simulink model "ridmasimulink"  (R2019b)
settings: Solver=VariableStepAuto  StartTime=0.0  StopTime=10.0  RelTol=1e-3
values from neighbouring files (symbols this model uses):
  A = [0 0 1 0 ... (first row only)    [RIP_ABCD_SS.m]    (also in RIP_ABCD_SS_1.m; RIP_ABCD_SS_2.m = [0   0    1   0; RIP_ABCD_SS_3.m; RIP_ABCD_SS_POLE_PLACE.m)
  B = Kg * kt * B / Rm    [RIP_ABCD_SS.m]    (also in RIP_ABCD_SS_1.m; RIP_ABCD_SS_2.m; RIP_ABCD_SS_3.m; RIP_ABCD_SS_POLE_PLACE.m)
  C = eye(2,4)    [RIP_ABCD_SS.m]    (also in RIP_ABCD_SS_1.m; RIP_ABCD_SS_2.m = [1 0 0 0; RIP_ABCD_SS_3.m; RIP_ABCD_SS_POLE_PLACE.m)
  D = zeros(2,1)    [RIP_ABCD_SS.m]    (also in RIP_ABCD_SS_1.m; RIP_ABCD_SS_2.m = [0; RIP_ABCD_SS_3.m; RIP_ABCD_SS_POLE_PLACE.m)
  K = [0 0 0 0]    [Pole_placement.m]    (also in RIP_ABCD_SS.m = lqr(A,B,Q,R); RIP_ABCD_SS_POLE_PLACE.m = lqr(A,B,Q,R); ripbalanced.m = acker(A,B,DP); setup_rotpen.m = d_balance(A, B, zeta, wn, p3, p4))
libraries: simulink_extras x3
settings Model: Creator=Ridma  LastModifiedBy=Ridma

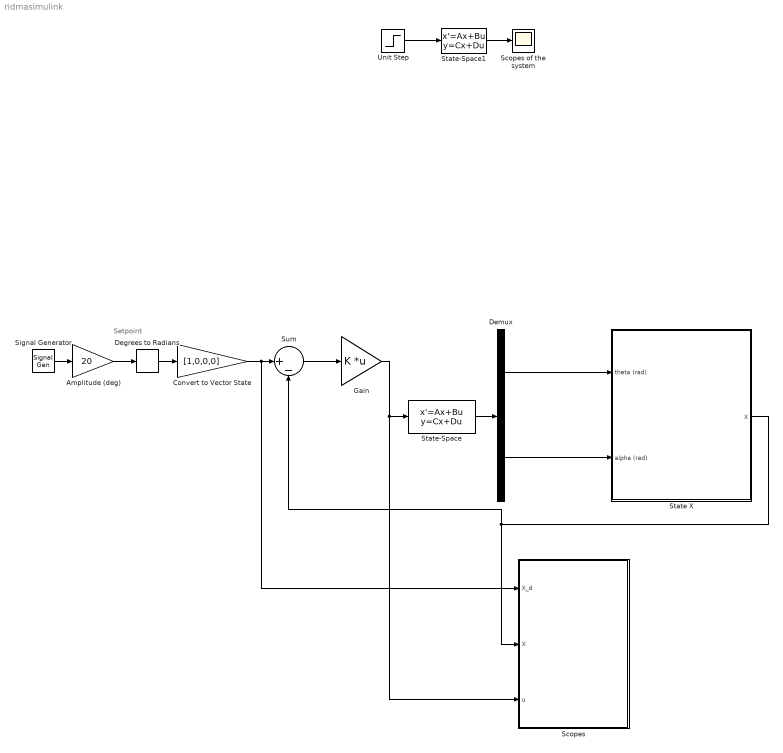
== system ridmasimulink ==
  note: Setpoint
  " State X " : Subsystem
      mask Display: image('$imagefile'); % Use "Edit Image" on toolstrip to change.
  Amplitude (deg) : Gain  Gain=20  SaturateOnIntegerOverflow=on  OutDataTypeStr=Inherit: Same as input  ParamDataTypeStr=Inherit: Same as input
  Convert to Vector State : Gain  Gain=[1,0,0,0]
  Degrees to Radians : simulink_extras/Transformations/Degrees to Radians
  Demux : Demux  Outputs=2
  Gain : Gain  Gain=K  Multiplication=Matrix(K*u)
  Scopes : Subsystem
  Scopes of the system : Scope
  Signal Generator : SignalGenerator  WaveForm=square  Frequency=0.1
  State-Space : StateSpace  A=A  B=B  C=C  D=D  InitialCondition=0
  State-Space1 : StateSpace  A=A  B=B  C=C  D=D  InitialCondition=0
  Sum : Sum  Inputs=|+-
  Unit Step : Step  SampleTime=0
  wires:
  Demux/2 -> " State X "/2(alpha (rad))
  Demux/1 -> " State X "/1(theta (rad))
  State-Space/1 -> Demux/1
  Amplitude (deg)/1 -> Degrees to Radians/1
  Degrees to Radians/1 -> Convert to Vector State/1
  Signal Generator/1 -> Amplitude (deg)/1
  Convert to Vector State/1 -> Scopes/1(X_d), Sum/1
  Sum/1 -> Gain/1
  Gain/1 -> Scopes/3(u), State-Space/1
  " State X "/1(X) -> Sum/2, Scopes/2(X)
  Unit Step/1 -> State-Space1/1
  State-Space1/1 -> Scopes of the system/1

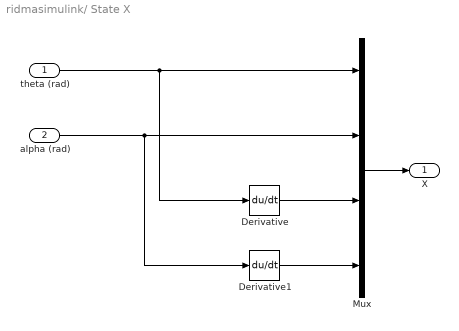
== system ridmasimulink/ State X  ==
  theta (rad) : Inport
  alpha (rad) : Inport  Port=2
  Derivative : Derivative
  Derivative1 : Derivative
  Mux : Mux
  X : Outport  VectorParamsAs1DForOutWhenUnconnected=off
  wires:
  alpha (rad)/1 -> Derivative1/1, Mux/2
  Mux/1 -> X/1
  theta (rad)/1 -> Derivative/1, Mux/1
  Derivative/1 -> Mux/3
  Derivative1/1 -> Mux/4

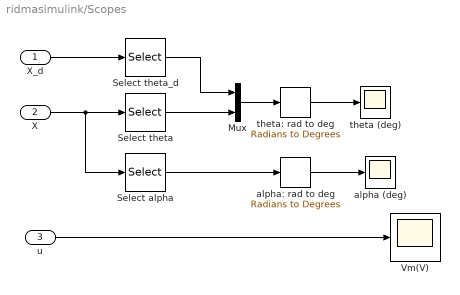
== system ridmasimulink/Scopes ==
  X_d : Inport
  X : Inport  Port=2
  u : Inport  Port=3
  Mux : Mux  Inputs=2
  Select alpha : Selector  InputPortWidth=4  IndexOptions=Index vector (dialog)  Indices=2  OutputSizes=[(-2)]
  Select theta : Selector  InputPortWidth=4  IndexOptions=Index vector (dialog)  Indices=1  OutputSizes=[(-2)]
  Select theta_d : Selector  InputPortWidth=4  IndexOptions=Index vector (dialog)  Indices=1  OutputSizes=[(-2)]
  Vm(V) : Scope
  alpha (deg) : Scope
  alpha: rad to deg : simulink_extras/Transformations/Radians to Degrees
  theta (deg) : Scope
  theta: rad to deg : simulink_extras/Transformations/Radians to Degrees
  wires:
  X_d/1 -> Select theta_d/1
  Select alpha/1 -> alpha: rad to deg/1
  X/1 -> Select alpha/1, Select theta/1
  Select theta_d/1 -> Mux/1
  Select theta/1 -> Mux/2
  u/1 -> Vm(V)/1
  alpha: rad to deg/1 -> alpha (deg)/1
  Mux/1 -> theta: rad to deg/1
  theta: rad to deg/1 -> theta (deg)/1
